simulink model "modelisation1"  (R2016b)
settings: Solver=VariableStepAuto  StartTime=0.0  StopTime=20  MaxStep=0.01  RelTol=1e-3
settings Model: Creator=BOUDOT  LastModifiedBy=BOUDOT

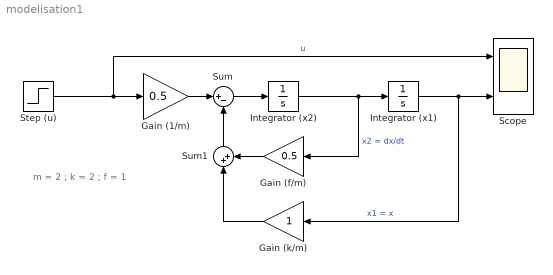
== system modelisation1 ==
  note: m = 2 ; k = 2 ; f = 1
  Gain (1/m) : Gain  Gain=0.5
  Gain (f/m) : Gain  Gain=0.5
  Gain (k/m) : Gain
  Integrator (x1) : Integrator
  Integrator (x2) : Integrator
  Scope : Scope  NumInputPorts=2
  Step (u) : Step  SampleTime=0
  Sum : Sum  Inputs=|+-
  Sum1 : Sum  Inputs=|++
  wires:
  Integrator (x2)/1 -> Integrator (x1)/1, Gain (f/m)/1  "x2 = dx/dt"
  Integrator (x1)/1 -> Gain (k/m)/1, Scope/2  "x1 = x"
  Step (u)/1 -> Scope/1, Gain (1/m)/1  "u"
  Sum/1 -> Integrator (x2)/1
  Sum1/1 -> Sum/2
  Gain (f/m)/1 -> Sum1/2
  Gain (1/m)/1 -> Sum/1
  Gain (k/m)/1 -> Sum1/1
